simulink model "VOO"  (R2022a)
settings: Solver=FixedStepAuto  StartTime=0.0  StopTime=10.0  FixedStep=1e-3  RelTol=1e-3  EnableMultiTasking=on
undefined symbols (not defined in the file or in its folder): D10, D11, D12, D2, D4, D5, D7, D8, D9, PTA0, PTA2, PTB23, PTB9, PTC3, PTC4, PTD0, PTD2, PTD3
libraries: frdmk64flib x9
settings Model: ExtModeTrigDuration=5  Creator=cathe  LastModifiedBy=anand
settings OptimizationCC: EnhancedBackFolding=on  PassReuseOutputArgsAs=Individual arguments  ZeroExternalMemoryAtStartup=off  ZeroInternalMemoryAtStartup=off  MaxStackSize=64  OptimizeBlockOrder=speed  DifferentSizesBufferReuse=on  OptimizationCustomize=off  EfficientTunableParamExpr=on
settings DebuggingCC: ParameterTunabilityLossMsg=error
settings HardwareCC: ProdBitPerPointer=32  ProdBitPerSizeT=32  ProdBitPerPtrDiffT=32  ProdLargestAtomicInteger=Long  ProdLargestAtomicFloat=Double  ProdWordSize=32  ProdHWDeviceType=ARM Compatible->ARM Cortex
settings SFSimCC: MATLABDynamicMemAlloc=off
settings RTWCC: SystemTargetFile=ert.tlc  HardwareBoard=NXP FRDM-K64F  TLCOptions="-aInlineSetEventsForThisBaseRateFcn=TLC_FALSE -aSuppressMultiTaskScheduler=TLC_FALSE  -aRateBasedStepFcn=0"  TemplateMakefile=ert_default_tmf  Toolchain=GNU Tools for ARM Embedded Processors
settings CodeAppCC: ForceParamTrailComments=on  IgnoreCustomStorageClasses=off  OperatorAnnotations=on  SimulinkDataObjDesc=on  SFDataObjDesc=on  InsertBlockDesc=on
settings ERTTargetCC: ExtModeTransport=4  ExtModeMexFile=sendToCommService

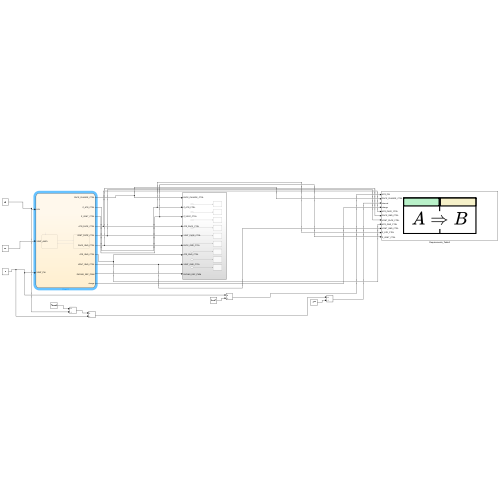
[thumbnail: Simulink's stored preview of the top-level diagram]
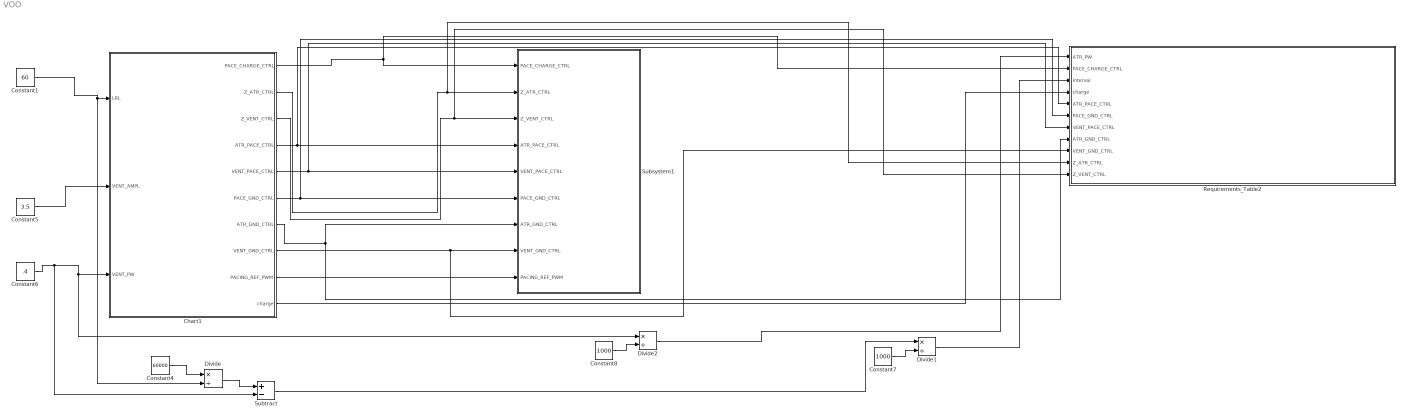
== system VOO ==
  Chart1 : Stateflow chart  TreatAsAtomicUnit=on
  Constant1 : Constant  Value=60
  Constant4 : Constant  Value=60000
  Constant5 : Constant  Value=3.5
  Constant6 : Constant  Value=.4
  Constant7 : Constant  Value=1000
  Constant8 : Constant  Value=1000
  Divide : Product  Inputs=*/
  Divide1 : Product  Inputs=*/
  Divide2 : Product  Inputs=*/
  Requirements_Table2 : Requirements Table  TreatAsAtomicUnit=on
  Subsystem1 : Subsystem
  Subtract : Sum  Inputs=+-
  wires:
  Subtract/1 -> Divide1/1
  Constant4/1 -> Divide/1
  Chart1/7(ATR_GND_CTRL) -> Requirements_Table2/8(ATR_GND_CTRL), Subsystem1/7(ATR_GND_CTRL)
  Constant1/1 -> Divide/2, Chart1/1(LRL)
  Chart1/5(VENT_PACE_CTRL) -> Requirements_Table2/7(VENT_PACE_CTRL), Subsystem1/5(VENT_PACE_CTRL)
  Chart1/10(charge) -> Requirements_Table2/4(charge)
  Chart1/6(PACE_GND_CTRL) -> Requirements_Table2/6(PACE_GND_CTRL), Subsystem1/6(PACE_GND_CTRL)
  Chart1/9(PACING_REF_PWM) -> Subsystem1/9(PACING_REF_PWM)
  Constant6/1 -> Subtract/2, Chart1/3(VENT_PW), Divide2/1
  Chart1/4(ATR_PACE_CTRL) -> Requirements_Table2/5(ATR_PACE_CTRL), Subsystem1/4(ATR_PACE_CTRL)
  Chart1/3(Z_VENT_CTRL) -> Requirements_Table2/11(Z_VENT_CTRL), Subsystem1/3(Z_VENT_CTRL)
  Divide/1 -> Subtract/1
  Constant8/1 -> Divide2/2
  Divide2/1 -> Requirements_Table2/1(ATR_PW)
  Divide1/1 -> Requirements_Table2/3(interval)
  Constant7/1 -> Divide1/2
  Chart1/1(PACE_CHARGE_CTRL) -> Requirements_Table2/2(PACE_CHARGE_CTRL), Subsystem1/1(PACE_CHARGE_CTRL)
  Chart1/8(VENT_GND_CTRL) -> Requirements_Table2/9(VENT_GND_CTRL), Subsystem1/8(VENT_GND_CTRL)
  Chart1/2(Z_ATR_CTRL) -> Requirements_Table2/10(Z_ATR_CTRL), Subsystem1/2(Z_ATR_CTRL)
  Constant5/1 -> Chart1/2(VENT_AMPL)

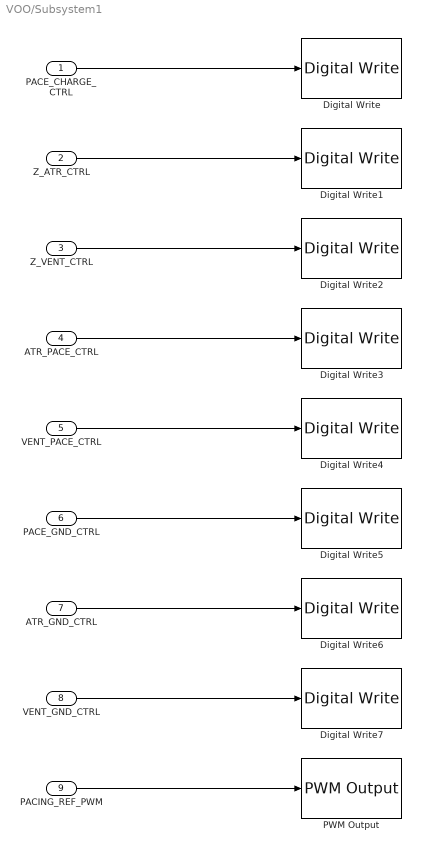
== system VOO/Subsystem1 ==
  PACE_CHARGE_CTRL : Inport
  Z_ATR_CTRL : Inport  Port=2
  Z_VENT_CTRL : Inport  Port=3
  ATR_PACE_CTRL : Inport  Port=4
  VENT_PACE_CTRL : Inport  Port=5
  PACE_GND_CTRL : Inport  Port=6
  ATR_GND_CTRL : Inport  Port=7
  VENT_GND_CTRL : Inport  Port=8
  PACING_REF_PWM : Inport  Port=9
  Digital Write : frdmk64flib/Digital Write  Whichpin=PTB9 (D2)
  Digital Write1 : frdmk64flib/Digital Write  Whichpin=PTB23 (D4)
  Digital Write2 : frdmk64flib/Digital Write  Whichpin=PTC3 (D7)
  Digital Write3 : frdmk64flib/Digital Write  Whichpin=PTA0 (D8)
  Digital Write4 : frdmk64flib/Digital Write  Whichpin=PTC4 (D9)
  Digital Write5 : frdmk64flib/Digital Write  Whichpin=PTD0 (D10)
  Digital Write6 : frdmk64flib/Digital Write  Whichpin=PTD2 (D11)
  Digital Write7 : frdmk64flib/Digital Write  Whichpin=PTD3 (D12)
  PWM Output : frdmk64flib/PWM Output  Whichpin=PTA2 (D5)  InitialFrequency=2000  InitialDutyCycle=0
  wires:
  PACE_CHARGE_CTRL/1 -> Digital Write/1
  Z_ATR_CTRL/1 -> Digital Write1/1
  Z_VENT_CTRL/1 -> Digital Write2/1
  ATR_PACE_CTRL/1 -> Digital Write3/1
  VENT_PACE_CTRL/1 -> Digital Write4/1
  PACE_GND_CTRL/1 -> Digital Write5/1
  ATR_GND_CTRL/1 -> Digital Write6/1
  VENT_GND_CTRL/1 -> Digital Write7/1
  PACING_REF_PWM/1 -> PWM Output/1

== stateflow chart VOO/Chart1 ==
  state CHARGING_DISCHARGING
    entry:
    charge = true;
    %DISCHARGING C21
    PACE_GND_CTRL = true;
    VENT_PACE_CTRL = false;
    Z_ATR_CTRL = false;
    Z_VENT_CTRL = false;
    ATR_PACE_CTRL = false;
    ATR_GND_CTRL = true;
    VENT_GND_CTRL = false;
    %CHARGING C22
    PACING_REF_PWM = 100*VENT_AMPL/5;
    PACE_CHARGE_CTRL = true;
  state PACE_ATR
    entry:
    charge = false;
    PACE_CHARGE_CTRL = false;
    PACE_GND_CTRL = true;
    ATR_PACE_CTRL = false;
    ATR_GND_CTRL = false;
    Z_ATR_CTRL = false;
    Z_VENT_CTRL = false;
    VENT_GND_CTRL = false;
    VENT_PACE_CTRL = true;
  (default) -> CHARGING_DISCHARGING
  CHARGING_DISCHARGING -> PACE_ATR : [after(60000/LRL-VENT_PW, msec)]
  PACE_ATR -> CHARGING_DISCHARGING : [after(VENT_PW,msec)]
  data: LRL input; PACE_CHARGE_CTRL output; Z_ATR_CTRL output; Z_VENT_CTRL output; ATR_PACE_CTRL output; VENT_PACE_CTRL output; PACE_GND_CTRL output; ATR_GND_CTRL output; VENT_GND_CTRL output; PACING_REF_PWM output; charge output boolean; VENT_AMPL input; VENT_PW input

== stateflow chart VOO/Requirements_Table2 ==
  (default) -> (junction 1073742982)
  (junction 1073742982) -> (junction 1073742983) : {
      | % SF_REQ_REV_07
      | }
  (junction 1073742983) -> (junction 1073742985) : {
      | % HEADER_ASSIGNMENTS
      |
      | }
  (junction 1073742985) -> (junction 1073742987) : {
      | % START_A_4
      | }
  (junction 1073742987) -> (junction 1073742989) : {
      | }
  (junction 1073742989) -> (junction 1073742991)
  (junction 1073742991) -> (junction 1073742993) : {
      | }
  (junction 1073742993) -> (junction 1073742995) : {
      | % END_A_4
      | }
  (junction 1073742995) -> (junction 1073742997) : {
      | % START_R_16
      | }
  (junction 1073742997) -> (junction 1073742999) : {
      | }
  (junction 1073742999) -> (junction 1073743001)
  (junction 1073743001) -> (junction 1073743003) [order 1] : [(charge == true && t<(interval))]
  (junction 1073743001) -> (junction 1073743009) [order 2]
  (junction 1073743003) -> (junction 1073743005) : {
      | reqtable_postcondition((PACE_GND_CTRL == true && VENT_PACE_CTRL == false && Z_ATR_CTRL == false && Z_VENT_CTRL == false && ATR_PACE_CTRL == false && ATR_GND_CTRL == true && VENT_GND_CTRL == false && PACE_CHARGE_CTRL == true ), 'R:1');
      |
      |
      | }
  (junction 1073743005) -> (junction 1073743007) : {
      | }
  (junction 1073743007) -> (junction 1073743009)
  (junction 1073743009) -> (junction 1073743011)
  (junction 1073743011) -> (junction 1073743013) : {
      | % END_R_16
      | }
  (junction 1073743013) -> (junction 1073743015) : {
      | % START_R_19
      | }
  (junction 1073743015) -> (junction 1073743017) : {
      | }
  (junction 1073743017) -> (junction 1073743019)
  (junction 1073743019) -> (junction 1073743021) [order 1] : [( charge == false && (interval)<=t<= (interval+ATR_PW))]
  (junction 1073743019) -> (junction 1073743027) [order 2]
  (junction 1073743021) -> (junction 1073743023) : {
      | reqtable_postcondition((PACE_CHARGE_CTRL == false && PACE_GND_CTRL == true && PACE_GND_CTRL == true && VENT_PACE_CTRL == true && Z_ATR_CTRL == false && Z_VENT_CTRL == false && ATR_PACE_CTRL == false && ATR_GND_CTRL == false && VENT_GND_CTRL == false), 'R:2');
      |
      |
      | }
  (junction 1073743023) -> (junction 1073743025) : {
      | }
  (junction 1073743025) -> (junction 1073743027)
  (junction 1073743027) -> (junction 1073743029)
  (junction 1073743029) -> (junction 1073743031) : {
      | % END_R_19
      | }
  (junction 1073743031) -> (junction 1073743033) : {
      | % START_R_13
      | }
  (junction 1073743033) -> (junction 1073743035) : {
      | }
  (junction 1073743035) -> (junction 1073743037)
  (junction 1073743037) -> (junction 1073743039) [order 1] : [( charge == true && t > interval)]
  (junction 1073743037) -> (junction 1073743045) [order 2]
  (junction 1073743039) -> (junction 1073743041) : {
      | reqtable_postcondition((PACE_GND_CTRL == true && VENT_PACE_CTRL == false && Z_ATR_CTRL == false && Z_VENT_CTRL == false && ATR_PACE_CTRL == false && ATR_GND_CTRL == true && VENT_GND_CTRL == false && PACE_CHARGE_CTRL == true ), 'R:3');
      |
      |
      | }
  (junction 1073743041) -> (junction 1073743043) : {
      | }
  (junction 1073743043) -> (junction 1073743045)
  (junction 1073743045) -> (junction 1073743047)
  (junction 1073743047) -> (junction 1073743049) : {
      | % END_R_13
      | }
  data: ATR_PW input double; PACE_CHARGE_CTRL input; interval input; charge input boolean; ATR_PACE_CTRL input boolean; PACE_GND_CTRL input boolean; VENT_PACE_CTRL input boolean; ATR_GND_CTRL input boolean; VENT_GND_CTRL input boolean; Z_ATR_CTRL input boolean; Z_VENT_CTRL input boolean
